simulink model "MRACsim"  (R2019a)
settings: Solver=VariableStepAuto  StartTime=0.0  StopTime=300  RelTol=1e-3
values from neighbouring files (symbols this model uses):
  a0 = 3    [Gradient_instant_cost.m]    (also in Gradient_integral_cost.m; MRAC.m = 3+n(1); MRAC2.m = 1+n(1); MRAC3.m = 1)
  a1 = 2    [Gradient_instant_cost.m]    (also in Gradient_integral_cost.m; MRAC.m = 5+n(2); MRAC2.m = 5+n(2); MRAC3.m = 3)
  b0 = 1    [Gradient_instant_cost.m]    (also in Gradient_integral_cost.m; MRAC.m = 7+n(3); MRAC2.m = 3+n(3); MRAC3.m = 3)
  beta = 1    [Untitled9.m]
  gamma = diag([0.01,0.01,0.005,0.005])    [MRAC3.m]    (also in Parameter_estimation.m = 10*i; Untitled2.m = 10; Untitled34.m = 1; Untitled9.m = 1)
  lambda = [lambda1; lambda0]    [Gradient_instant_cost.m]    (also in Gradient_integral_cost.m; PureLSQ.m; Untitled2.m = 10; Untitled34.m = 1)
  w0 = 3    [MRAC.m]    (also in MRAC2.m; Untitled2.m = 1; Untitled5.m = 2; Untitled9.m = 1)
  zeta = 1    [MRAC.m]    (also in MRAC2.m; Untitled5.m; Untitled9.m)
settings Model: Creator=Student  LastModifiedBy=Student

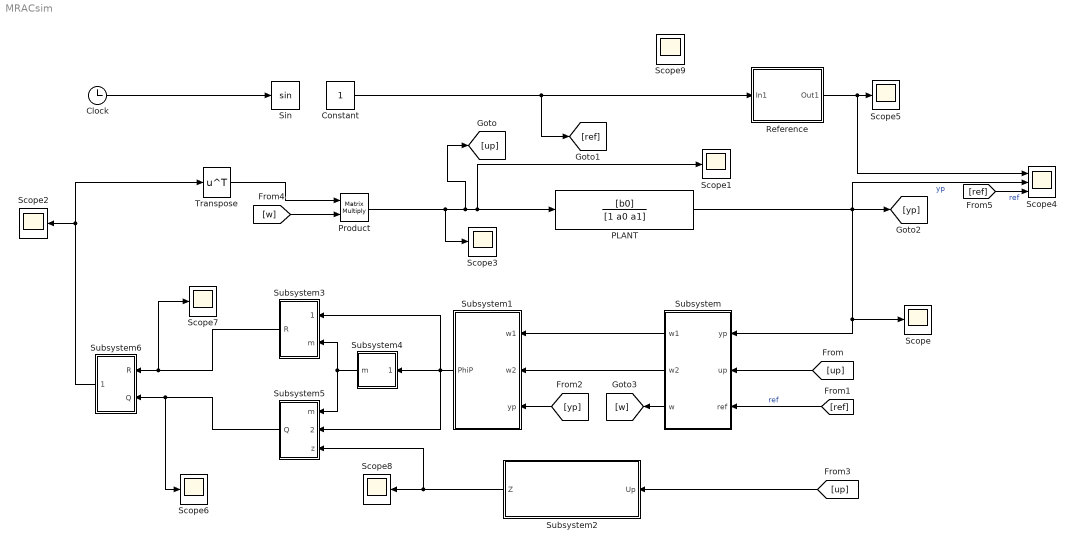
== system MRACsim ==
  Clock : Clock
  Constant : Constant
  PLANT : TransferFcn  Numerator=[b0]  Denominator=[1 a0 a1]
  Product : Product  Multiplication=Matrix(*)
  Reference : Subsystem
  Scope{,1..3,5..9} (9 alike) : Scope
  Scope4 : Scope  NumInputPorts=3
  Sin : Trigonometry
  Subsystem : Subsystem
  Subsystem1 : Subsystem
  Subsystem2 : Subsystem
  Subsystem3 : Subsystem
  Subsystem4 : Subsystem
  Subsystem5 : Subsystem
  Subsystem6 : Subsystem
  Transpose : Math  Operator=transpose  SaturateOnIntegerOverflow=on
  wires:
  Reference/1(Out1) -> Scope4/1, Scope5/1
  PLANT/1 -> Scope/1, Subsystem/1(yp), Scope4/2, [yp]  "yp"
  [up] -> Subsystem/2("up ")
  [ref] -> Subsystem/3(ref)  "ref"
  Subsystem/1(w1) -> Subsystem1/1(w1)
  Subsystem/2("w2 ") -> Subsystem1/2(w2)
  [yp] -> Subsystem1/3(yp)
  [up] -> Subsystem2/1(Up)
  Subsystem/3("w ") -> [w]
  Subsystem1/1(PhiP) -> Subsystem5/2("Phip "), Subsystem4/1(Phip), Subsystem3/1("Phip ")
  Subsystem4/1(m) -> Subsystem5/1("m "), Subsystem3/2("m ")
  Subsystem2/1(Z) -> Scope8/1, Subsystem5/3(z)
  Subsystem3/1(R) -> Scope7/1, Subsystem6/1("R ")
  Subsystem5/1(Q) -> Scope6/1, Subsystem6/2(Q)
  Transpose/1 -> Product/1
  Subsystem6/1(Theta) -> Scope2/1, Transpose/1
  Product/1 -> Scope3/1, Scope1/1, PLANT/1, [up]
  Clock/1 -> Sin/1
  [w] -> Product/2
  [ref] -> Scope4/3  "ref"
  Constant/1 -> [ref], Reference/1(In1)

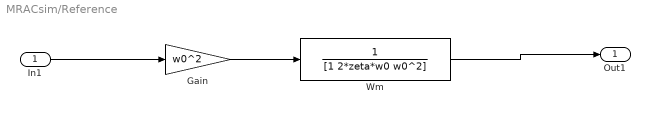
== system MRACsim/Reference ==
  In1 : Inport
  Gain : Gain  Gain=w0^2
  "Wm " : TransferFcn  Denominator=[1 2*zeta*w0 w0^2]
  Out1 : Outport
  wires:
  Gain/1 -> "Wm "/1
  In1/1 -> Gain/1
  "Wm "/1 -> Out1/1

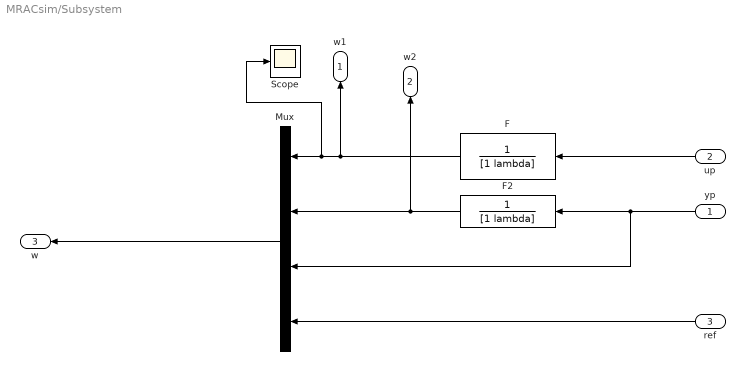
== system MRACsim/Subsystem ==
  yp : Inport
  "up " : Inport  Port=2
  ref : Inport  Port=3
  F : TransferFcn  Denominator=[1 lambda]
  F2 : TransferFcn  Denominator=[1 lambda]
  Mux : Mux
  Scope : Scope
  w1 : Outport
  "w2 " : Outport  Port=2
  "w " : Outport  Port=3
  wires:
  "up "/1 -> F/1
  F2/1 -> "w2 "/1, Mux/2
  F/1 -> Scope/1, Mux/1, w1/1
  Mux/1 -> "w "/1
  ref/1 -> Mux/4
  yp/1 -> Mux/3, F2/1

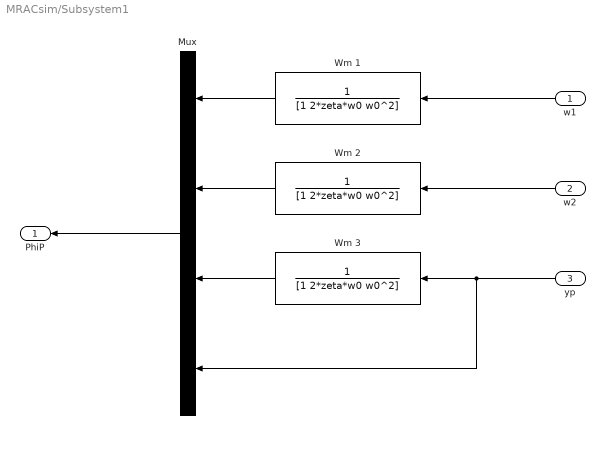
== system MRACsim/Subsystem1 ==
  w1 : Inport
  w2 : Inport  Port=2
  yp : Inport  Port=3
  Mux : Mux
  Wm 1 : TransferFcn  Denominator=[1 2*zeta*w0 w0^2]
  Wm 2 : TransferFcn  Denominator=[1 2*zeta*w0 w0^2]
  Wm 3 : TransferFcn  Denominator=[1 2*zeta*w0 w0^2]
  PhiP : Outport
  wires:
  yp/1 -> Mux/4, Wm 3/1
  Wm 2/1 -> Mux/2
  Wm 3/1 -> Mux/3
  w1/1 -> Wm 1/1
  Mux/1 -> PhiP/1
  Wm 1/1 -> Mux/1
  w2/1 -> Wm 2/1

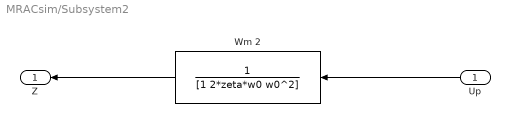
== system MRACsim/Subsystem2 ==
  Up : Inport
  Wm 2 : TransferFcn  Denominator=[1 2*zeta*w0 w0^2]
  Z : Outport
  wires:
  Up/1 -> Wm 2/1
  Wm 2/1 -> Z/1

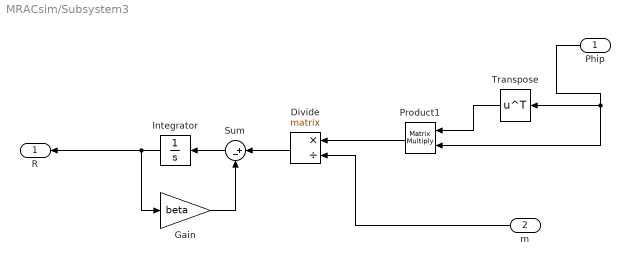
== system MRACsim/Subsystem3 ==
  "Phip " : Inport
  "m " : Inport  Port=2
  Divide : Product  Inputs=*/  Multiplication=Matrix(*)
  Gain : Gain  Gain=beta
  Integrator : Integrator  InitialCondition=[0,0,0,0;0,0,0,0;0,0,0,0;0,0,0,0]
  Product1 : Product  Multiplication=Matrix(*)
  Sum : Sum  Inputs=|+-
  Transpose : Math  Operator=transpose  SaturateOnIntegerOverflow=on
  R : Outport
  wires:
  Gain/1 -> Sum/2
  Integrator/1 -> Gain/1, R/1
  Sum/1 -> Integrator/1
  "m "/1 -> Divide/2
  Divide/1 -> Sum/1
  Product1/1 -> Divide/1
  "Phip "/1 -> Product1/2, Transpose/1
  Transpose/1 -> Product1/1

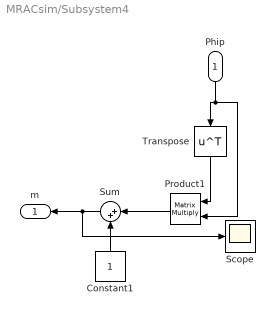
== system MRACsim/Subsystem4 ==
  Phip : Inport
  Constant1 : Constant
  Product1 : Product  Multiplication=Matrix(*)
  Scope : Scope
  Sum : Sum  Inputs=|++
  Transpose : Math  Operator=transpose  SaturateOnIntegerOverflow=on
  m : Outport
  wires:
  Constant1/1 -> Sum/2
  Product1/1 -> Sum/1
  Phip/1 -> Transpose/1, Product1/2
  Sum/1 -> Scope/1, m/1
  Transpose/1 -> Product1/1

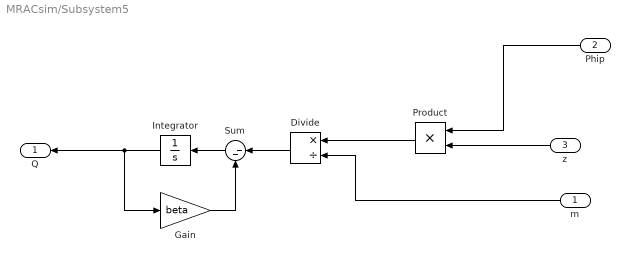
== system MRACsim/Subsystem5 ==
  "m " : Inport
  "Phip " : Inport  Port=2
  z : Inport  Port=3
  Divide : Product  Inputs=*/
  Gain : Gain  Gain=beta
  Integrator : Integrator  InitialCondition=[0;0;0;0]
  Product : Product
  Sum : Sum  Inputs=|--
  Q : Outport
  wires:
  Gain/1 -> Sum/2
  "Phip "/1 -> Product/1
  Integrator/1 -> Gain/1, Q/1
  Sum/1 -> Integrator/1
  "m "/1 -> Divide/2
  Divide/1 -> Sum/1
  Product/1 -> Divide/1
  z/1 -> Product/2

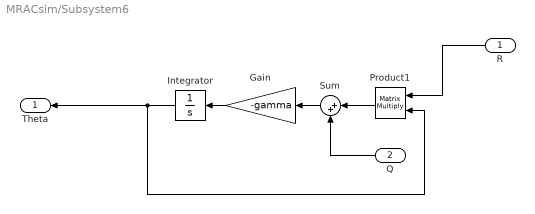
== system MRACsim/Subsystem6 ==
  "R " : Inport
  Q : Inport  Port=2
  Gain : Gain  Gain=-gamma
  Integrator : Integrator  InitialCondition=[1,1,1,1]
  Product1 : Product  Multiplication=Matrix(*)
  Sum : Sum  Inputs=|++
  Theta : Outport
  wires:
  Gain/1 -> Integrator/1
  Sum/1 -> Gain/1
  Q/1 -> Sum/2
  Integrator/1 -> Product1/2, Theta/1
  Product1/1 -> Sum/1
  "R "/1 -> Product1/1
